simulink model "DEA_c"  (R2018a)
settings: Solver=ode15s  StartTime=0.0  StopTime=100  EnableMultiTasking=on
InitFcn:
  | Parameter;
settings Model: Creator=Johannes  LastModifiedBy=Matthias
settings DataIOCC: LimitDataPoints=on  SaveFormat=Array  SignalLoggingSaveFormat=ModelDataLogs
settings OptimizationCC: LifeSpan=inf
settings DebuggingCC: UnderspecifiedInitializationDetection=Classic  MergeDetectMultiDrivingBlocksExec=none  SolverPrmCheckMsg=warning  MultiTaskDSMMsg=warning  MultiTaskCondExecSysMsg=none  SFUnexpectedBacktrackingDiag=warning  SFNoUnconditionalDefaultTransitionDiag=warning  SFExecutionAtInitializationDiag=none
settings HardwareCC: ProdBitPerPointer=32  ProdBitPerSizeT=32  ProdBitPerPtrDiffT=32  ProdLargestAtomicFloat=None  ProdIntDivRoundTo=Undefined  ProdEndianess=Unspecified  ProdWordSize=32  ProdHWDeviceType=32-bit Generic
settings ModelReferenceCC: PropagateSignalLabelsOutOfModel=off
settings CodeAppCC: StateflowObjectComments=on
settings GRTTargetCC: TargetLangStandard=C89/C90 (ANSI)  GeneratePreprocessorConditionals=Disable all
settings ConfigComp: CovMetricSettings=dw  CovHtmlReporting=on  CovSaveCumulativeToWorkspaceVar=on  CovSaveSingleToWorkspaceVar=on  CovExternalEMLEnable=off

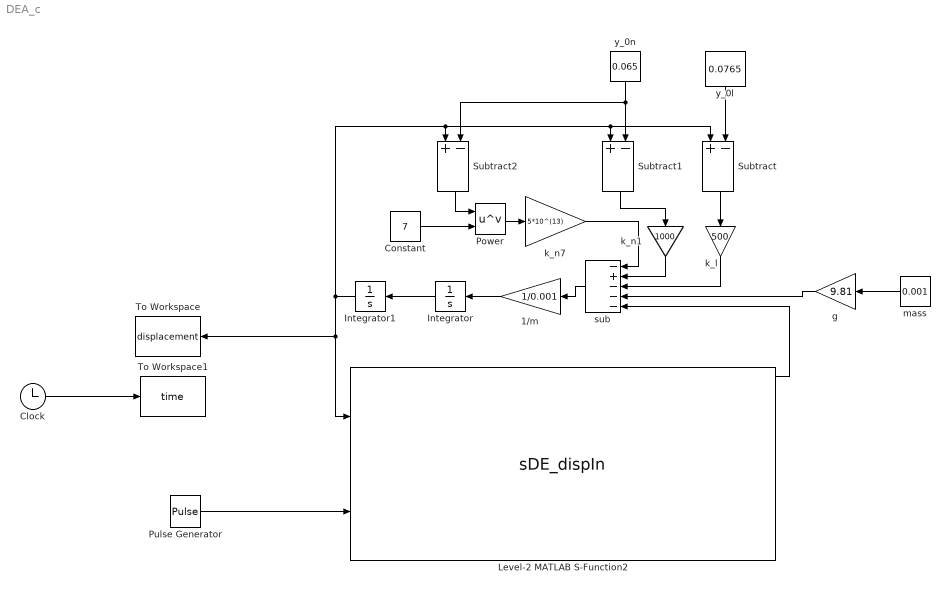
== system DEA_c ==
  1/m : Gain  Gain=1/0.001
  Clock : Clock
  Constant : Constant  Value=7
  Integrator : Integrator
  Integrator1 : Integrator  InitialCondition=0.053
  Level-2 MATLAB S-Function2 : M-S-Function  FunctionName=sDE_dispIn  Parameters=params, initConds
      mask Display:
      | color('black');
      | patch(4*[-1 1 1 -1],1.75*[-1 -1 1 1],[1 1 1]);
      | patch(2*[-1 1 1 -1],1.2*[-1 -1 1 1],[0 0 0]);
      | patch(1.95*[-1 1 1 -1],0.8*[-1 -1 1 1],[1 1 1]);
      | disp('DE Actuator');
      | 
      | color('blue');
      | port_label('input', 1, 'y [m]','texmode','on');
      | port_label('input', 2, 'v [V]','texmode','on');
      | 
      | color('red');
      | port_label('output', 1, 'F [N]','texmode','on');
      | port_label('output', 2, 'x_v [-]','texmode','on');
      | port_label('output', 3, 'q [C]','texmode','on');
      | port_label('output', 4, '\epsilon_1 [-]','texmode','on');
      | port_label('output', 5, '\sigma_1 [Pa]','texmode','on');
      | port_label('output', 6, 'i [A]','texmode','on');
      | port_label('output', 7, 'v_{DE} [V]','texmode','on');
      | port_label('output', 8, 'C [F]','texmode','on');
  Power : Math  Operator=pow  SaturateOnIntegerOverflow=on
  Pulse Generator : DiscretePulseGenerator  PulseType=Time based  Amplitude=2500  Period=10  PulseWidth=50
  Subtract : Sum  Inputs=+-
  Subtract1 : Sum  Inputs=+-
  Subtract2 : Sum  Inputs=+-
  To Workspace : ToWorkspace  VariableName=displacement  SampleTime=-1
  To Workspace1 : ToWorkspace  VariableName=time  SampleTime=-1
  g : Gain  Gain=9.81
  k_l : Gain  Gain=500
  k_n1 : Gain  Gain=1000
  k_n7 : Gain  Gain=5*10^(13)
  mass : Constant  Value=0.001
  sub : Sum  Inputs=-+---
  "y_0l " : Constant  Value=0.0765
  y_0n : Constant  Value=0.065
  wires:
  1/m/1 -> Integrator/1
  Integrator/1 -> Integrator1/1
  mass/1 -> g/1
  sub/1 -> 1/m/1
  "y_0l "/1 -> Subtract/2
  Subtract/1 -> k_l/1
  Level-2 MATLAB S-Function2/1 -> sub/5
  g/1 -> sub/4
  k_l/1 -> sub/3
  y_0n/1 -> Subtract1/2, Subtract2/2
  Subtract1/1 -> k_n1/1
  k_n1/1 -> sub/2
  Power/1 -> k_n7/1
  k_n7/1 -> sub/1
  Pulse Generator/1 -> Level-2 MATLAB S-Function2/2
  Integrator1/1 -> Subtract1/1, Subtract/1, Subtract2/1, To Workspace/1, Level-2 MATLAB S-Function2/1
  Clock/1 -> To Workspace1/1
  Subtract2/1 -> Power/1
  Constant/1 -> Power/2
